simulink model "MSFartoystyring_heading_controller"  (R2018a)
settings: Solver=ode45  StartTime=tstart  StopTime=tstop  RelTol=1e-3  EnableMultiTasking=on
values from neighbouring files (symbols this model uses):
  c = 0    [run_heading.m]    (also in run_heading_controller.m = 1; run_heading_model.m; run_path.m; run_path_crab.m)
  K_d = 2*zeta*w_n*(m + K_m) - d    [run_heading_controller.m]
  K_i = w_n / 10 * K_p    [run_heading_controller.m]
  K_p = (m+K_m)*w_n^2 - k    [run_heading_controller.m]
  p0 = zeros(2,1)    [run_heading.m]    (also in run_heading_controller.m; run_heading_model.m; run_path.m = [1000; 700]; run_path_crab.m = [1000; 700])
  psi0 = 0    [run_heading.m]    (also in run_heading_controller.m; run_heading_model.m; run_path.m = deg2rad(-135); run_path_crab.m = deg2rad(-135))
  psi_d0 = deg2rad(15)    [run_heading_controller.m]    (also in run_speed_controller.m = deg2rad(0))
  psi_d_A = 0.4    [run_heading_controller.m]    (also in run_speed_controller.m)
  psi_d_w = 0.004    [run_heading_controller.m]    (also in run_speed_controller.m)
  r0 = 0    [run_heading.m]    (also in run_heading_controller.m; run_heading_model.m; run_path.m; run_path_crab.m)
  T_step = 3000    [run_heading_controller.m]    (also in run_heading_model.m; run_speed_controller.m)
  tsamp = 10    [run_heading.m]    (also in run_heading_controller.m = 1; run_heading_model.m = 1; run_path.m = 1; run_path_crab.m)
  v0 = [6.63 0]'    [run_heading.m]    (also in run_heading_controller.m; run_heading_model.m; run_path.m; run_path_crab.m)
undefined symbols (not defined in the file or in its folder): msfartoystyring
settings Model: ExtModeAutoUpdateStatusClock=off  Creator=christh  LastModifiedBy=nicho
settings DataIOCC: LimitDataPoints=on  SaveFormat=Array  SignalLoggingSaveFormat=ModelDataLogs
settings OptimizationCC: ExpressionDepthLimit=2147483647  InitFltsAndDblsToZero=on  LifeSpan=inf
settings DebuggingCC: UnderspecifiedInitializationDetection=Classic  MergeDetectMultiDrivingBlocksExec=none  SolverPrmCheckMsg=warning  FcnCallInpInsideContextMsg=warning  StateNameClashWarn=warning  SFUnexpectedBacktrackingDiag=warning  SFNoUnconditionalDefaultTransitionDiag=warning  SFExecutionAtInitializationDiag=none
settings HardwareCC: ProdBitPerPointer=32  ProdBitPerSizeT=32  ProdBitPerPtrDiffT=32  ProdLargestAtomicFloat=None  ProdIntDivRoundTo=Undefined  ProdEndianess=Unspecified  ProdWordSize=32  ProdHWDeviceType=32-bit Generic
settings ModelReferenceCC: PropagateSignalLabelsOutOfModel=off
settings CodeAppCC: StateflowObjectComments=on
settings GRTTargetCC: TargetLangStandard=C89/C90 (ANSI)  GeneratePreprocessorConditionals=Disable all  CombineOutputUpdateFcns=off  GRTInterface=on
settings ConfigComp: CovMetricSettings=dw  CovHtmlReporting=on  CovSaveCumulativeToWorkspaceVar=on  CovSaveSingleToWorkspaceVar=on  CovExternalEMLEnable=off

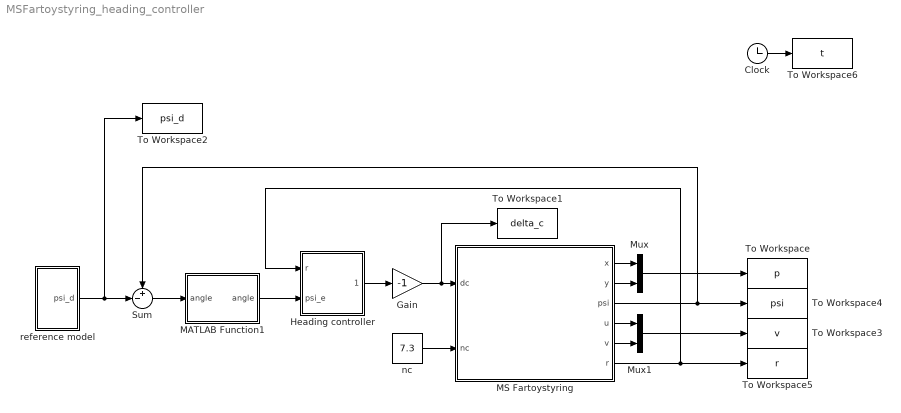
== system MSFartoystyring_heading_controller ==
  Clock : Clock
  Gain : Gain  Gain=-1
  Heading controller : Subsystem
  MATLAB Function1 : MATLAB Function  TreatAsAtomicUnit=on
  MS Fartoystyring : Subsystem  mask(MS Fartoystyring for Assignment 3 G&C){x0=p0(1), y0=p0(2), u0=v0(1), v0=v0(2), psi0=psi0, r0=r0, c=c}
      mask prompts: x0 "x(t0) (m)"; y0 "y(t0) (m)"; u0 "u(t0) (m/s)"; v0 "v(t0) (m/s)"; psi0 "psi(t0) (rad)"; r0 "r(t0) (rad/s)"; c "current (0 or 1)"
      mask help:
      | Block corresponding to Figure 1 in the assignment text. Gives the response of the ship.
      |
      | The design speed of MS Fartoystyring is u=8.23 m/s.
      |
      | Input:
      | dc: commanded rudder (rad), dmax=25*pi/180
      | nc: commanded shaft speed (rad/s), nmax=85*2*pi/60
      |
      | Output:
      | x: north pos (m)
      | y: east pos (m)
      | u: surge (m/s)
      | v: sway (m/s)
      | psi: heading (rad)
      | r: yaw (rad/s)
      mask Help: Comments, bugs and help requests can be directed to the TA. Email on course website.
  Mux : Mux  Inputs=2
  Mux1 : Mux  Inputs=2
  Sum : Sum  Inputs=+-|
  To Workspace : ToWorkspace  VariableName=p  SampleTime=tsamp
  To Workspace1 : ToWorkspace  VariableName=delta_c  SampleTime=tsamp
  To Workspace2 : ToWorkspace  VariableName=psi_d  SampleTime=tsamp
  To Workspace3 : ToWorkspace  VariableName=v  SampleTime=tsamp
  To Workspace4 : ToWorkspace  VariableName=psi  SampleTime=tsamp
  To Workspace5 : ToWorkspace  VariableName=r  SampleTime=tsamp
  To Workspace6 : ToWorkspace  VariableName=t  SampleTime=tsamp
  nc : Constant  Value=7.3
  reference model : Subsystem
  wires:
  Clock/1 -> To Workspace6/1
  MS Fartoystyring/1(x) -> Mux/1
  MS Fartoystyring/2(y) -> Mux/2
  MS Fartoystyring/4(u) -> Mux1/1
  MS Fartoystyring/5(v) -> Mux1/2
  Mux/1 -> To Workspace/1
  Mux1/1 -> To Workspace3/1
  MS Fartoystyring/6(r) -> Heading controller/1(r), To Workspace5/1
  nc/1 -> MS Fartoystyring/2(nc)
  Heading controller/1(delta_c) -> Gain/1
  MS Fartoystyring/3(psi) -> Sum/1, To Workspace4/1
  reference model/1(psi_d) -> To Workspace2/1, Sum/2
  Sum/1 -> MATLAB Function1/1("angle ")
  MATLAB Function1/1(angle) -> Heading controller/2(psi_e)
  Gain/1 -> To Workspace1/1, MS Fartoystyring/1(dc)

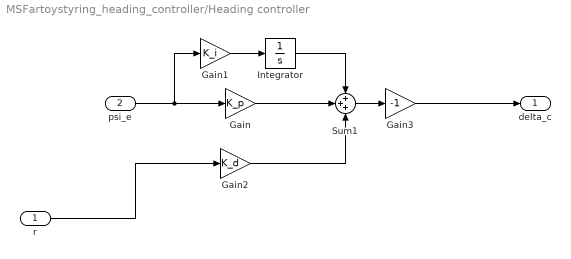
== system MSFartoystyring_heading_controller/Heading controller ==
  r : Inport
  psi_e : Inport  Port=2
  Gain : Gain  Gain=K_p
  Gain1 : Gain  Gain=K_i
  Gain2 : Gain  Gain=K_d
  Gain3 : Gain  Gain=-1
  Integrator : Integrator
  Sum1 : Sum  Inputs=+++
  delta_c : Outport
  wires:
  Integrator/1 -> Sum1/1
  Gain2/1 -> Sum1/3
  Gain1/1 -> Integrator/1
  Gain/1 -> Sum1/2
  psi_e/1 -> Gain1/1, Gain/1
  r/1 -> Gain2/1
  Sum1/1 -> Gain3/1
  Gain3/1 -> delta_c/1

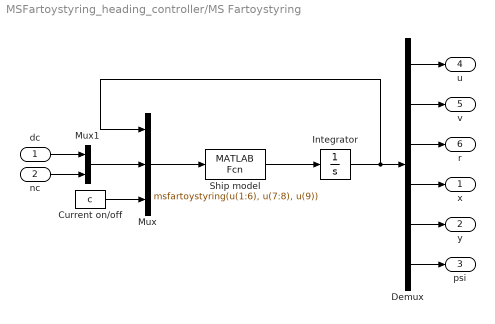
== system MSFartoystyring_heading_controller/MS Fartoystyring ==
  dc : Inport
  nc : Inport  Port=2
  Current on/off : Constant  Value=c
  Demux : Demux  Outputs=6
  Integrator : Integrator  InitialCondition=[u0 v0 r0 x0 y0 psi0]'
  Mux : Mux  Inputs=3
  Mux1 : Mux  Inputs=2
  Ship model : MATLABFcn  MATLABFcn=msfartoystyring(u(1:6), u(7:8), u(9))  OutputDimensions=6
  x : Outport
  y : Outport  Port=2
  psi : Outport  Port=3
  u : Outport  Port=4
  v : Outport  Port=5
  r : Outport  Port=6
  wires:
  Integrator/1 -> Mux/1, Demux/1
  Mux1/1 -> Mux/2
  dc/1 -> Mux1/1
  nc/1 -> Mux1/2
  Demux/1 -> u/1
  Demux/2 -> v/1
  Demux/3 -> r/1
  Demux/4 -> x/1
  Demux/5 -> y/1
  Demux/6 -> psi/1
  Current on/off/1 -> Mux/3
  Ship model/1 -> Integrator/1
  Mux/1 -> Ship model/1

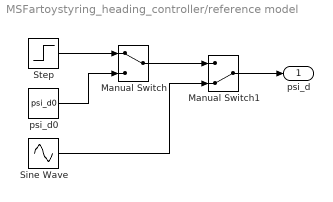
== system MSFartoystyring_heading_controller/reference model ==
  Manual Switch : ManualSwitch
  Manual Switch1 : ManualSwitch  CurrentSetting=0
  Sine Wave : Sin  Amplitude=psi_d_A  Frequency=psi_d_w  SampleTime=0
  Step : Step  Time=T_step  After=psi_d0  SampleTime=0
  psi_d0 : Constant  Value=psi_d0
  psi_d : Outport
  wires:
  psi_d0/1 -> Manual Switch/2
  Step/1 -> Manual Switch/1
  Sine Wave/1 -> Manual Switch1/2
  Manual Switch/1 -> Manual Switch1/1
  Manual Switch1/1 -> psi_d/1

== matlab function MSFartoystyring_heading_controller/MATLAB Function1 ==
  data: angle input; angle output
function angle = ssa(angle)
    angle = mod(angle + pi, 2*pi) - pi;
